simulink model "s_cd_hmc_v3_pol0"  (R2016b)
(part 13 of 31)

  Gateway Out59/1 -> To Workspace72/1
  bus_expand5/5(out4) -> Gateway Out59/1
  Gateway Out62/1 -> To Workspace73/1
  bus_expand5/6(out3) -> Gateway Out62/1
  Gateway Out63/1 -> To Workspace74/1
  bus_expand5/7(out2) -> Gateway Out63/1
  Gateway Out64/1 -> To Workspace77/1
  bus_expand5/8(lsb_out1) -> Gateway Out64/1
  Slice6/1 -> bus_expand5/1(bus_in)
  Gateway Out72/1 -> To Workspace47/1
  Gateway Out73/1 -> To Workspace46/1
  Gateway Out66/1 -> To Workspace48/1
  bus_expand6/3(out6) -> Gateway Out66/1
  bus_expand6/2(out7) -> Gateway Out73/1
  bus_expand6/1(msb_out8) -> Gateway Out72/1
  Gateway Out67/1 -> To Workspace49/1
  bus_expand6/4(out5) -> Gateway Out67/1
  Gateway Out68/1 -> To Workspace59/1
  bus_expand6/5(out4) -> Gateway Out68/1
  Gateway Out69/1 -> To Workspace60/1
  bus_expand6/6(out3) -> Gateway Out69/1
  Gateway Out70/1 -> To Workspace67/1
  bus_expand6/7(out2) -> Gateway Out70/1
  Gateway Out71/1 -> To Workspace68/1
  bus_expand6/8(lsb_out1) -> Gateway Out71/1
  Slice5/1 -> bus_expand6/1(bus_in)
  Gateway Out75/1 -> To Workspace69/1
  [hmc_reord_data] -> Slice5/1, Slice6/1, Gateway Out74/1
  Gateway Out74/1 -> To Workspace81/1
  Gateway Out76/1 -> To Workspace82/1
  Gateway Out77/1 -> To Workspace83/1
  Gateway Out88/1 -> To Workspace98/1
  bus_expand7/3(out6) -> Gateway Out78/1
  bus_expand7/2(out7) -> Gateway Out100/1
  bus_expand7/1(msb_out8) -> Gateway Out88/1
  bus_expand7/4(out5) -> Gateway Out79/1
  bus_expand7/5(out4) -> Gateway Out80/1
  bus_expand7/6(out3) -> Gateway Out81/1
  bus_expand7/7(out2) -> Gateway Out86/1
  bus_expand7/8(lsb_out1) -> Gateway Out87/1
  Gateway Out98/1 -> To Workspace85/1
  Gateway Out99/1 -> To Workspace86/1
  Gateway Out89/1 -> To Workspace89/1
  bus_expand8/3(out6) -> Gateway Out89/1
  bus_expand8/2(out7) -> Gateway Out99/1
  bus_expand8/1(msb_out8) -> Gateway Out98/1
  Gateway Out90/1 -> To Workspace90/1
  bus_expand8/4(out5) -> Gateway Out90/1
  Gateway Out92/1 -> To Workspace94/1
  bus_expand8/5(out4) -> Gateway Out92/1
  Gateway Out94/1 -> To Workspace95/1
  bus_expand8/6(out3) -> Gateway Out94/1
  Gateway Out95/1 -> To Workspace96/1
  bus_expand8/7(out2) -> Gateway Out95/1
  Gateway Out97/1 -> To Workspace97/1
  bus_expand8/8(lsb_out1) -> Gateway Out97/1
  Gateway Out78/1 -> To Workspace99/1
  Gateway Out79/1 -> To Workspace100/1
  Gateway Out80/1 -> To Workspace101/1
  Gateway Out81/1 -> To Workspace102/1
  Gateway Out86/1 -> To Workspace103/1
  Gateway Out87/1 -> To Workspace104/1
  Gateway Out100/1 -> To Workspace105/1
  Slice7/1 -> bus_expand8/1(bus_in)
  Slice8/1 -> bus_expand7/1(bus_in)
  Gateway Out119/1 -> To Workspace115/1
  bus_expand9/3(out6) -> Gateway Out102/1
  bus_expand9/2(out7) -> Gateway Out101/1
  bus_expand9/1(msb_out8) -> Gateway Out119/1
  bus_expand9/4(out5) -> Gateway Out103/1
  bus_expand9/5(out4) -> Gateway Out104/1
  bus_expand9/6(out3) -> Gateway Out105/1
  bus_expand9/7(out2) -> Gateway Out115/1
  bus_expand9/8(lsb_out1) -> Gateway Out118/1
  Gateway Out102/1 -> To Workspace107/1
  Gateway Out103/1 -> To Workspace109/1
  Gateway Out104/1 -> To Workspace112/1
  Gateway Out105/1 -> To Workspace114/1
  Gateway Out115/1 -> To Workspace116/1
  Gateway Out118/1 -> To Workspace117/1
  Gateway Out101/1 -> To Workspace106/1
  Slice9/1 -> bus_expand9/1(bus_in)
  Delay9/1 -> [hmc_reord_dvalid], Gateway Out180/1
  Gateway Out120/1 -> To Workspace84/1
  Gateway Out121/1 -> To Workspace118/1
  Reorder_cntrl/2(bram_rd_en) -> Delay9/1, [reord_bram_en_pol0], Gateway Out7/1, HMC_reord_bram/7
  [sys_rst] -> Logical11/3
